simulink model "DAbstractOperations"  (Simulink 7.8)
settings: Solver=ode45  StartTime=0.0  StopTime=10.0  RelTol=1e-3
settings Model: Creator=ah875096  LastModifiedBy=Deng

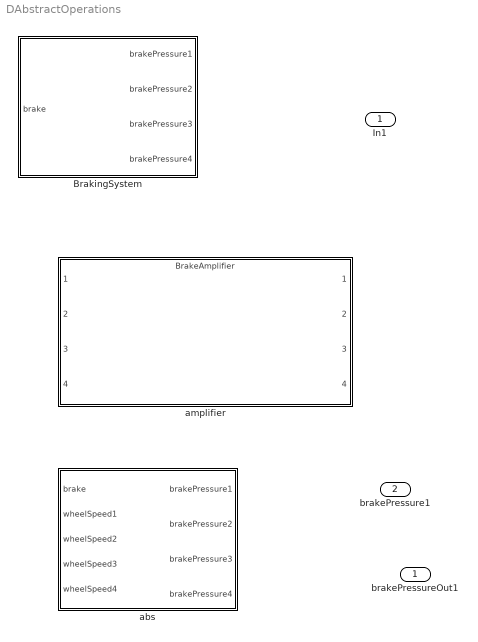
== system DAbstractOperations ==
  In1 : Inport
  BrakingSystem : Subsystem  TreatAsAtomicUnit=on
  abs : Subsystem  TreatAsAtomicUnit=on
  amplifier : ModelReference  ModelNameDialog=BrakeAmplifier  SimulationMode=Normal  ModelReferenceVersion=1.5  CopyOfModelName=BrakeAmplifier  DefaultDataLogging=on
  brakePressureOut1 : Outport
  brakePressure1 : Outport  Port=2

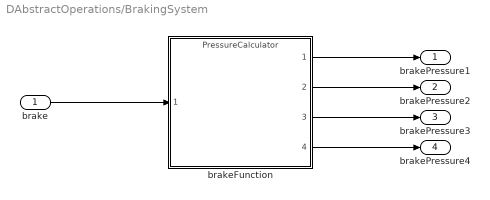
== system DAbstractOperations/BrakingSystem ==
  brake : Inport
  brakeFunction : ModelReference  ModelNameDialog=PressureCalculator  SimulationMode=Normal  ModelReferenceVersion=1.5  CopyOfModelName=PressureCalculator  DefaultDataLogging=on
  brakePressure1 : Outport
  brakePressure2 : Outport  Port=2
  brakePressure3 : Outport  Port=3
  brakePressure4 : Outport  Port=4
  wires:
  brake/1 -> brakeFunction/1
  brakeFunction/1 -> brakePressure1/1
  brakeFunction/2 -> brakePressure2/1
  brakeFunction/4 -> brakePressure4/1
  brakeFunction/3 -> brakePressure3/1

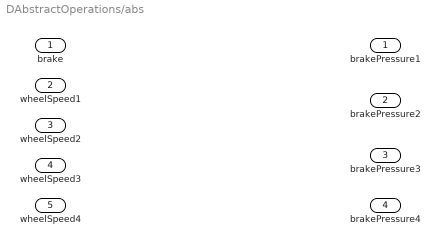
== system DAbstractOperations/abs ==
  brake : Inport
  wheelSpeed1 : Inport  Port=2
  wheelSpeed2 : Inport  Port=3
  wheelSpeed3 : Inport  Port=4
  wheelSpeed4 : Inport  Port=5
  brakePressure1 : Outport
  brakePressure2 : Outport  Port=2
  brakePressure3 : Outport  Port=3
  brakePressure4 : Outport  Port=4
